simulink model "GI"  (R2019a)
settings: Solver=VariableStepAuto  StartTime=0.0  StopTime=10.0  RelTol=1e-3
undefined symbols (not defined in the file): Q_gG, R_GGU, V_gG
settings Model: Creator=jcp2  LastModifiedBy=jcp2

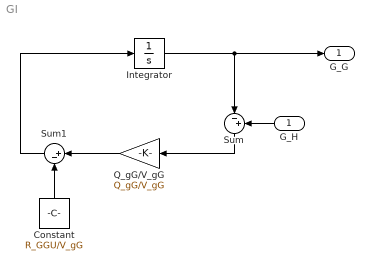
== system GI ==
  G_H : Inport
  Constant : Constant  Value=R_GGU/V_gG
  Integrator : Integrator
  Q_gG/V_gG : Gain  Gain=Q_gG/V_gG
  Sum : Sum  Inputs=|-+
  Sum1 : Sum  Inputs=|+-
  G_G : Outport
  wires:
  Integrator/1 -> G_G/1, Sum/1
  Q_gG/V_gG/1 -> Sum1/1
  G_H/1 -> Sum/2
  Sum/1 -> Q_gG/V_gG/1
  Constant/1 -> Sum1/2
  Sum1/1 -> Integrator/1
